simulink model "RockySimulink"  (R2021a)
settings: Solver=VariableStepAuto  StartTime=0.0  StopTime=10.0  RelTol=1e-3
values from neighbouring files (symbols this model uses):
  K = 0.00273    [RockySimulinkVars.m]
  Ki = 9.197759550739140e+03    (= 9197.75955074)    [RockySimulinkVars.m]
  Kp = 1.068233097931057e+03 + 1.159126922089819e-69    (= 1068.23309793)    [RockySimulinkVars.m]
  l = 0.456    [RockySimulinkVars.m]
undefined symbols (not defined in the file or in its folder): Tau
settings Model: Creator=mtong1  LastModifiedBy=mtong1

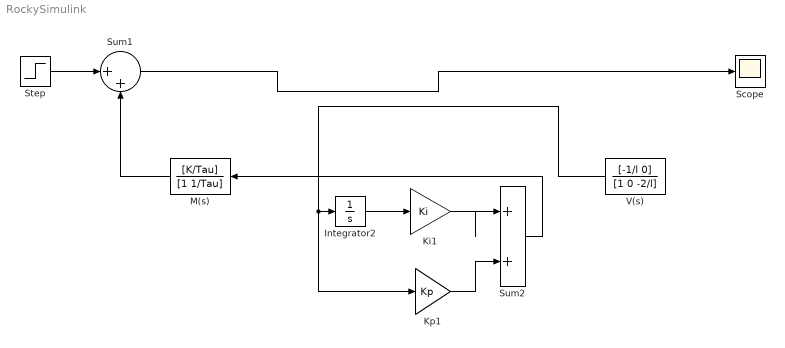
== system RockySimulink ==
  Integrator2 : Integrator
  Ki1 : Gain  Gain=Ki
  Kp1 : Gain  Gain=Kp
  M(s) : TransferFcn  Numerator=[K/Tau]  Denominator=[1 1/Tau]
  Scope : Scope
  Step : Step  After=20  SampleTime=0
  Sum1 : Sum  Inputs=|++
  Sum2 : Sum  Inputs=|++
  V(s) : TransferFcn  Numerator=[-1/l 0]  Denominator=[1 0 -2/l]
  wires:
  Step/1 -> Sum1/1
  M(s)/1 -> Sum1/2
  Integrator2/1 -> Ki1/1
  V(s)/1 -> Kp1/1, Integrator2/1
  Ki1/1 -> Sum2/1
  Kp1/1 -> Sum2/2
  Sum2/1 -> M(s)/1
  Sum1/1 -> Scope/1
